simulink model "Algebraicka_slucka"  (R2018b)
settings: Solver=VariableStepAuto  StartTime=0.0  StopTime=10.0  RelTol=1e-3
settings Model: Creator=domin  LastModifiedBy=domin

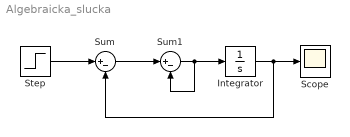
== system Algebraicka_slucka ==
  Integrator : Integrator
  Scope : Scope
  Step : Step  SampleTime=0
  Sum : Sum  Inputs=|+-
  Sum1 : Sum  Inputs=|+-
  wires:
  Step/1 -> Sum/1
  Sum/1 -> Sum1/1
  Sum1/1 -> Sum1/2, Integrator/1
  Integrator/1 -> Sum/2, Scope/1
